simulink model "Link_A_org"  (Simulink 10.0)
settings: Solver=FixedStepAuto  StartTime=0  StopTime=15  FixedStep=1  RelTol=1e-3
StopFcn:
  | %set_param(gcb,'TAP_R_INI',[num2str(Tap_pu_R(end)), '  %Updated']);
libraries: simulink x9
(part 1 of 2)
settings Model: Creator=aw5670  LastModifiedBy=annonymous
settings DataIOCC: LimitDataPoints=on
settings OptimizationCC: BlockReduction=off  BooleanDataType=off
settings DebuggingCC: SaveWithParameterizedLinksMsg=none  SignalResolutionControl=TryResolveAllWithWarning
settings HardwareCC: TargetUnknown=on
settings GRTTargetCC: GeneratePreprocessorConditionals=Disable all  CombineOutputUpdateFcns=on  GRTInterface=off
settings ConfigComp: CovExternalEMLEnable=off  CovSFcnEnable=off

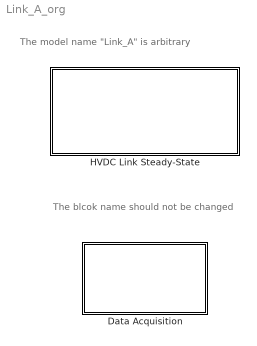
== system Link_A_org ==
  note: The blcok name should not be changed
  note: The model name "Link_A" is arbitrary
  Data Acquisition : Subsystem  mask{Ts=1}
      mask prompts: Ts "Sample time :"
      mask Display: disp('Open this block\nto visualize\nrecorded signals')
  HVDC Link Steady-State : Subsystem  mask(HVDC link steady-state model){NB_R=2, NOT_USED_3=, NOT_USED_4=, Pn_R=600, U1_R=[735, 0.0025, 0.01], U2_R=[200, 0.0025, 0.11], NOT_USED_0=DC current, NOT_USED_1=0, AMODE_ANGLE=5, LOCK_TAP_R=off, TCC_UDI0_MODE_R=off, ANGLE_R=[14.0, 17.0], Udi0_ref_R=280, TSTP_R=0.0125, TAP_R=[0.9375, 1.125], TAP_R_INI=0.9375  %Updated, Eac_R_INI=740.941  %Updated, NB_I=2, NOT_USED_5=, NOT_USED_6=, Pn_I=600, U1_I=[735, 0.0025, 0.01], U2_I=[200, 0.0025, 0.11], C_MODE_I=DC voltage, GAMMA_REF=22, VSCHED=500, GMODE_ANGLE=17, NOT_USED_2=0, LOCK_TAP_I=off, TCC_UDI0_MODE_I=off, ANGLE_I=[20.0, 23.0], Udi0_ref_I=280, TSTP_I=0.0125, TAP_I=[0.9125, 1.0875], TAP_I_INI=0.9875  %Updated, Eac_I_INI=759.4246  %Updated, RDC=12.0 + 2*0.3, RCOMP=0.3, MC_MODE=Power, SLACK_ST=Rectifier, SETVAL_MW=1000, SETVAL_kA=2, VCMODE=500*0.94, DELTI=0.2, Tap_pu_R=0.9375, Eac_R=740.8893, Udi0_R=290.4097, Tap_limited_R=0, alpha_R=16.1762, Idc_R=2, Vdc_R=524.6, Pdc_R=1049.2, Pac_R=1054.5333, Qac_R=479.4564, Tap_pu_I=0.975, Eac_I=758.8212, Udi0_I=285.9986, Tap_limited_I=0, alpha_I=144.587, gamma_I=22.8031, Vdc_I=499.4, Pdc_I=-998.8, Pac_I=-993.4667, Qac_I=562.6279, DC_iter=2, Ts=1}
      mask prompts: NB_R "Number of 6 pulse converter units in series"; NOT_USED_3 "AC bus name"; NOT_USED_4 "PQ load name"; Pn_R "Power (MVA)"; U1_R "Primary winding (AC side) parameters [V1 Ph-Ph(kVrms), R1(pu), L1(pu)]"; U2_R "Secondary winding (DC side) parameters [V2 Ph-Ph(kVrms), R2(pu), L2(pu)]"; NOT_USED_0 "Control mode"; NOT_USED_1 "not used"; AMODE_ANGLE "Minimum alpha (deg.)"; LOCK_TAP_R "Lock tap ratio"; TCC_UDI0_MODE_R "Udi0 control mode"; ANGLE_R "Angle range [min, max] (deg.)"; Udi0_ref_R "Udi0 reference (kV)"; TSTP_R "Tap step size (pu)"; TAP_R "Tap range [min, max] (pu)"; TAP_R_INI "Tap ratio (pu)"; Eac_R_INI "Primary AC voltage  (Ph-Ph(kVrms))"; NB_I "Number of 6 pulse converter units in series"; NOT_USED_5 "AC bus name"; NOT_USED_6 "PQ load name"; Pn_I "Power (MVA)"; U1_I "Primary winding (AC side) parameters [V1 Ph-Ph(kVrms), R1(pu), L1(pu)]"; U2_I "Secondary winding (DC side) parameters [V2 Ph-Ph(kVrms), R2(pu), L2(pu)]"; C_MODE_I "Control mode"; GAMMA_REF "Gamma reference (deg.)"; VSCHED "Voltage reference (kV)"; GMODE_ANGLE "Minimum gamma (deg.)"; NOT_USED_2 "Not used"; LOCK_TAP_I "Lock tap ratio"; TCC_UDI0_MODE_I "Udi0 control mode"; ANGLE_I "Angle range  [min, max] (deg.)"; Udi0_ref_I "Udi0 reference (kV)"; TSTP_I "Tap step size (pu)"; TAP_I "Tap range [min, max] (pu)"; TAP_I_INI "Tap ratio (pu)"; Eac_I_INI "Primary AC voltage  (Ph-Ph(kVrms))"; RDC "Total link resistance (ohm)"; RCOMP "Resistance between voltage measurement and converter (ohm)"; MC_MODE "Control mode"; SLACK_ST "Slack station"; SETVAL_MW "Power reference (MW)"; SETVAL_kA "Current reference (kA)"; VCMODE "Inverter DC voltage threshold in power control (kV)"; DELTI "Inverter current margin (kA)"; Tap_pu_R "Tap ratio (pu)"; Eac_R "Eac (kV)"; Udi0_R "Udi0 (kV)"; Tap_limited_R "Tap is limited"; alpha_R "Alpha (deg.)"; Idc_R "Idc (kA)"; Vdc_R "Vdc (kV)"; Pdc_R "Pdc (MW)"; Pac_R "Pac (MW)"; Qac_R "Qac (Mvar)"; Tap_pu_I "Tap ratio (pu)"; Eac_I "Eac (kV)"; Udi0_I "Udi0 (kV)"; Tap_limited_I "Tap is limited"; alpha_I "Alpha (deg.)"; gamma_I "Gamma (deg.)"; Vdc_I "Vdc (kV)"; Pdc_I "Pdc (MW)"; Pac_I "Pac (MW)"; Qac_I "Qac (Mvar)"; DC_iter "Iterations"; Ts "Sample time :"
      mask help: Implements a steady state model of a two terminal HVDC link for the DC load flow solution.
      mask init:
      | % History values 
      | Eac_R     = Eac_R_INI;
      | Eac_I     = Eac_I_INI;
      | TAPINI_R  = TAP_R_INI;
      | TAPINI_I  = TAP_I_INI;
      | 
      | % --- RECTIFIER ---
      | 
      | % Primary
      | V1_R = U1_R(1);
      | R1_R = U1_R(2);
      | L1_R = U1_R(3);
      | 
      | % Secondary
      | V2_R = U2_R(1);
      | R2_R = U2_R(2);
      | L2_R = U2_R(3);
      | 
      | % Nominal turn ratio (Usec/Uprim):
      | TR_R = V2_R/V1_R;
      | 
      | % Transformer reactance seen from secondary, per bridge [XC](ohm):
      | XC_R = (L1_R+L2_R)*V2_R^2/Pn_R;
      | 
      | % Transformer resistance seen from secondary, per bridge [RC](ohm):
      | RC_R = (R1_R+R2_R)* V2_R^2/Pn_R; 
      | 
      | % Tap Changer Control
      | ALFMIN_R=ANGLE_R(1);
      | ALFMAX_R=ANGLE_R(2);
      | 
      | TAPMN_R=TAP_R(1);
      | TAPMX_R=TAP_R(2);
      | 
      | % --- INVERTER ---
      | % Primary
      | V1_I = U1_I(1);
      | R1_I = U1_I(2);
      | L1_I = U1_I(3);
      | 
      | % Secondary
      | V2_I = U2_I(1);
      | R2_I = U2_I(2);
      | L2_I = U2_I(3);
      | 
      | % Nominal turn ratio (Usec/Uprim):
      | TR_I = V2_I/V1_I;
      | 
      | % Transformer reactance seen from secondary, per bridge [XC](ohm):
      | XC_I = (L1_I+L2_I)*V2_I^2/Pn_I;
      | 
      | % Transformer resistance seen from secondary, per bridge [RC](ohm):
      | RC_I = (R1_I+R2_I)* V2_I^2/Pn_I; 
      | 
      | % Pole Control
      | GC = C_MODE_I - 1;  % GC (0/1) is used in the model
      | 
      | % Tap Changer Control
      | GAMMIN_I=ANGLE_I(1);
      | GAMMAX_I=ANGLE_I(2);
      | 
      | TAPMN_I=TAP_I(1);
      | TAPMX_I=TAP_I(2);
      | 
      | DCVMIN_I   = VSCHED * (1 - TSTP_I);     %(kV)
      | DCVMAX_I   = VSCHED * (1 + TSTP_I);
      | 
      | %Udi0_min = (1-TSTP*0.75)* Udi0_ref;  % kV
      | %Udi0_max = (1+TSTP*0.75)* Udi0_ref;
      | 
      | % --- Master Control ---
      | MDC = MC_MODE - 1;     % MDC (0,1, or 2) used in the model 
      | 
      | if (MDC == 1)   
      |     SETVAL = SETVAL_MW;
      | elseif (MDC == 2)
      |     SETVAL = SETVAL_kA;
      | else
      |     SETVAL = 0;
      | end
      mask Help: web('HVDC_Link_SS_help.htm');
      mask TypeOptions NOT_USED_0: DC current
      mask Callback LOCK_TAP_R:
      | mode=get_param(gcb,'LOCK_TAP_R');
      | cb = get_param(gcb,'MaskEnables');
      | cb{11}='on'; cb{12}='on';
      | 
      | if strcmp(mode,'on')
      |  cb{11}='off';  % Udi0 control mode
      |  cb{12}='off';  % Angle range
      | end
      | 
      | set_param(gcb,'MaskEnables',cb);
      mask Callback TCC_UDI0_MODE_R:
      | mode=get_param(gcb,'TCC_UDI0_MODE_R');
      | cb = get_param(gcb,'MaskEnables');
      | cb{10}='on'; cb{12}='on'; cb{13}='off';
      | 
      | if strcmp(mode,'on')
      |  cb{12}='off';  % Angle range
      |  cb{10}='off';  % Lock the tap position
      |  cb{13}='on';  % Lock the tap position
      | end
      | 
      | set_param(gcb,'MaskEnables',cb);
      mask TypeOptions C_MODE_I: DC voltage | Gamma angle
      mask Callback C_MODE_I:
      | mode=get_param(gcb,'C_MODE_I');
      | cb = get_param(gcb,'MaskEnables');
      | cb{25}='on'; cb{26}='on'; cb{27}='on'; cb{31}='on';
      | 
      | if strcmp(mode,'Gamma angle')
      |  cb{26}='off';    % Voltage reference
      |  cb{27}='off';    % Minimum gamma
      |  cb{31}='off';    % Angle range (gamma_
      | else
      |  cb{25}='off';    % Gamma reference
      | end
      | 
      | set_param(gcb,'MaskEnables',cb);
      mask Callback LOCK_TAP_I:
      | mode=get_param(gcb,'LOCK_TAP_I');
      | cb = get_param(gcb,'MaskEnables');
      | cb{30}='on'; cb{31}='on';
      | 
      | if strcmp(mode,'on')
      |  cb{30}='off';  % Udi0 control mode
      |  cb{31}='off';  % Angle range
      | end
      | 
      | set_param(gcb,'MaskEnables',cb);
      mask Callback TCC_UDI0_MODE_I:
      | mode=get_param(gcb,'TCC_UDI0_MODE_I');
      | cb = get_param(gcb,'MaskEnables');
      | cb{29}='on'; cb{31}='on';  cb{32}='off';
      | 
      | if strcmp(mode,'on')
      |  cb{29}='off';  % Lock the tap position
      |  cb{31}='off';  % Angle range
      |  cb{32}='on';   % Udi0 reference
      | end
      | 
      | set_param(gcb,'MaskEnables',cb);
      mask TypeOptions MC_MODE: Blocked | Power | Current
      mask Callback MC_MODE:
      | mode=get_param(gcb,'MC_MODE');
      | cb = get_param(gcb,'MaskEnables');
      |  cb{40}='on'; cb{41}='on'; cb{42}='on'; cb{43}='on';
      | 
      | if strcmp(mode,'Current')
      |  cb{40}='off';     % Slack station
      |  cb{41}='off';     % Power reference
      |  cb{43}='off';     % Inverter DC ...
      | end
      | 
      | if strcmp(mode,'Power')
      |  cb{42}='off';     % Current reference
      | end
      | 
      | set_param(gcb,'MaskEnables',cb);
      | clear cb mode;
      mask TypeOptions SLACK_ST: Rectifier | Inverter
      mask DialogControl Update_tap_R Prompt: Update
      mask DialogControl Update_tap_R Callback:
      | set_param(gcb,'TAP_R_INI',[num2str(Tap_pu_R(end)), '  %Updated']);
      | 
      | % Reset output values
      | set_param(gcb,'Idc_R',[num2str(0)]);
      | set_param(gcb,'alpha_R',[num2str(0)]);
      | set_param(gcb,'Udi0_R',[num2str(0)]);
      | set_param(gcb,'Vdc_R',[num2str(0)]);
      | set_param(gcb,'Pac_R',[num2str(0)]);
      | set_param(gcb,'Qac_R',[num2str(0)]);
      | set_param(gcb,'Pdc_R',[num2str(0)]);
      mask DialogControl Update_tap_I Prompt: Update
      mask DialogControl Update_tap_I Callback:
      | set_param(gcb,'TAP_I_INI',[num2str(Tap_pu_I(end)), '  %Updated']);
      | 
      | % Reset output values
      | set_param(gcb,'gamma_I',[num2str(0)]);
      | set_param(gcb,'alpha_I',[num2str(0)]);
      | set_param(gcb,'Udi0_I',[num2str(0)]);
      | set_param(gcb,'Vdc_I',[num2str(0)]);
      | set_param(gcb,'Pdc_I',[num2str(0)]);
      | set_param(gcb,'Pac_I',[num2str(0)]);
      | set_param(gcb,'Qac_I',[num2str(0)]);
      mask DialogControl Container31 Prompt: Rectifier
      mask DialogControl Container33 Prompt: Inverter
      mask DialogControl Control4 Prompt: Compute and Update
      mask DialogControl Control4 Callback:
      | sim(gcs);
      | set_param(gcb,'DC_iter',[num2str(DC_iter(end))]);
      | % Rectifier
      | set_param(gcb,'Eac_R',[num2str(Eac_R(end))]);
      | set_param(gcb,'Tap_pu_R',[num2str(Tap_pu_R(end))]);
      | set_param(gcb,'Tap_limited_R',[num2str(Tap_limited_R(end))]);
      | set_param(gcb,'Idc_R',[num2str(Idc_R(end))]);
      | set_param(gcb,'alpha_R',[num2str(alpha_R(end))]);
      | set_param(gcb,'Udi0_R',[num2str(Udi0_R(end))]);
      | set_param(gcb,'Vdc_R',[num2str(Vdc_R(end))]);
      | set_param(gcb,'Pdc_R',[num2str(Pdc_R(end))]);
      | set_param(gcb,'Pac_R',[num2str(Pac_R(end))]);
      | set_param(gcb,'Qac_R',[num2str(Qac_R(end))]);
      | 
      | % Inverter
      | set_param(gcb,'Eac_I',[num2str(Eac_I(end))]);
      | set_param(gcb,'Tap_pu_I',[num2str(Tap_pu_I(end))]);
      | set_param(gcb,'Tap_limited_I',[num2str(Tap_limited_I(end))]);
      | set_param(gcb,'gamma_I',[num2str(gamma_I(end))]);
      | set_param(gcb,'alpha_I',[num2str(alpha_I(end))]);
      | set_param(gcb,'Udi0_I',[num2str(Udi0_I(end))]);
      | set_param(gcb,'Vdc_I',[num2str(Vdc_I(end))]);
      | set_param(gcb,'Pdc_I',[num2str(Pdc_I(end))]);
      | set_param(gcb,'Pac_I',[num2str(Pac_I(end))]);
      | set_param(gcb,'Qac_I',[num2str(Qac_I(end))]);
      mask Display: disp('Steady-state model\nof HVDC link\n\n(for DC load flow solution)')

== system Link_A_org/Data Acquisition ==
  note: Data acquisition
  Bus Selector : BusSelector  OutputSignals=Udi0
  Bus Selector1 : BusSelector  OutputSignals=Tap_pu,Tap_is_limited
  Bus Selector2 : BusSelector  OutputSignals=Tap_pu,Tap_is_limited
  Bus Selector3 : BusSelector  OutputSignals=alpha_deg,Qac,Pac,Eac
  Bus Selector4 : BusSelector  OutputSignals=Udi0,gamma_deg,Qac,Pac,Eac,alpha_deg
  Bus Selector6 : BusSelector  OutputSignals=Vdc_R,Vdc_I,Idc_R,Idc_I,Pdc_R,Pdc_I
  Bus Selector7 : BusSelector  OutputSignals=Io1,Io2
  DCLink : Scope  NumInputPorts=5
  INV : Scope  NumInputPorts=7
  Master : Scope  NumInputPorts=2
  REC : Scope  NumInputPorts=7
  Terminator : Terminator
  Terminator1 : Terminator
  wires:
  [m_TCC_R] -> Bus Selector2/1
  Bus Selector4/5 -> INV/7  "<Eac>"
  Bus Selector4/4 -> INV/6  "<Pac>"
  Bus Selector4/3 -> INV/5  "<Qac>"
  Bus Selector4/2 -> INV/4  "<gamma_deg>"
  Bus Selector4/1 -> INV/3  "<Udi0>"
  Bus Selector4/6 -> Terminator1/1  "<alpha_deg>"
  Bus Selector6/4 -> Terminator/1  "<Idc_I>"
  [m_dc_ntw] -> Bus Selector6/1
  [m_TCC_I] -> Bus Selector1/1
  [m_conv_I] -> Bus Selector4/1
  Bus Selector2/1 -> REC/1  "<Tap_pu>"
  Bus Selector6/1 -> DCLink/1  "<Vdc_R>"
  Bus Selector3/3 -> REC/6  "<Pac>"
  Bus Selector3/1 -> REC/4  "<alpha_deg>"
  Bus Selector3/2 -> REC/5  "<Qac>"
  [m_conv_R] -> Bus Selector3/1, Bus Selector/1
  Bus Selector/1 -> REC/3  "<Udi0>"
  [m_master] -> Bus Selector7/1
  Bus Selector7/1 -> Master/1  "<Io1>"
  Bus Selector7/2 -> Master/2  "<Io2>"
  Bus Selector2/2 -> REC/2  "<Tap_is_limited>"
  Bus Selector1/2 -> INV/2  "<Tap_is_limited>"
  Bus Selector6/2 -> DCLink/2  "<Vdc_I>"
  Bus Selector6/3 -> DCLink/3  "<Idc_R>"
  Bus Selector6/5 -> DCLink/4  "<Pdc_R>"
  Bus Selector6/6 -> DCLink/5  "<Pdc_I>"
  Bus Selector1/1 -> INV/1  "<Tap_pu>"
  Bus Selector3/4 -> REC/7  "<Eac>"

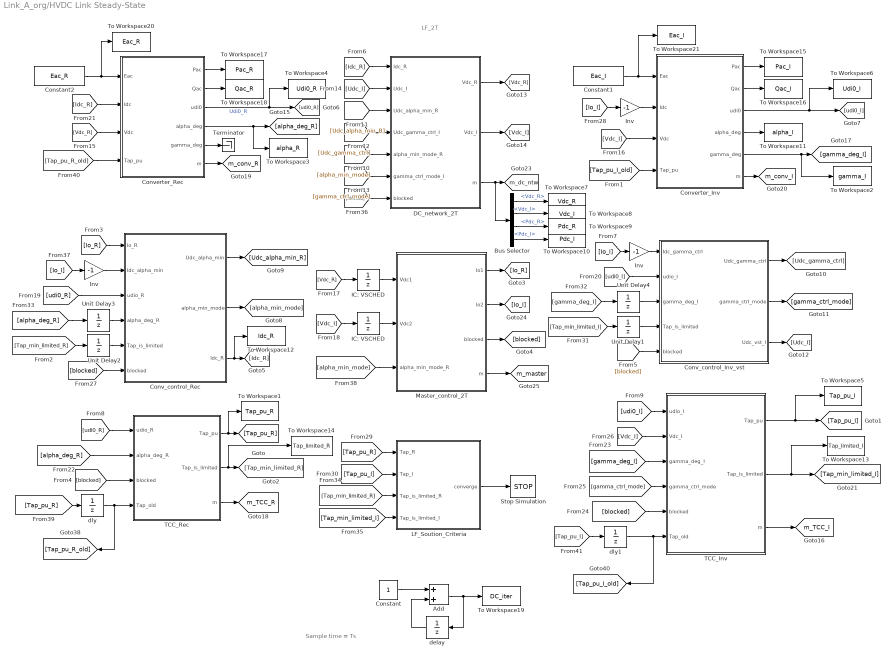
== system Link_A_org/HVDC Link Steady-State ==
  note: LF_2T
  note: Sample time = Ts
  " Inv " : Gain  Gain=-1
  Add : Sum
  Bus Selector : BusSelector  OutputSignals=Vdc_R,Vdc_I,Pdc_R,Pdc_I
  Constant : Constant
  Constant1 : Constant  Value=Eac_I
  Constant2 : Constant  Value=Eac_R
  Conv_control_Inv_vst : Subsystem  mask(Converter controls - voltage setting inverter){GC=GC, VSCHED=VSCHED, GMODE_ANGLE=GMODE_ANGLE, GAMMA_REF=GAMMA_REF, NB=NB_I, RC=RC_I, XC=XC_I}
      mask prompts: GC "Gamma control mode [GC] (1/0):"; VSCHED "Scheduled dc voltage [VSCHED] (kV):"; GMODE_ANGLE "Gamma minimum mode angle [GMODE_ANGLE] (deg):"; GAMMA_REF "Gamma reference angle [GAMMA_REF] (deg):"; NB "Number of 6 pulse bridges in series [NB]:"; RC "Resistance seen from secondary, per bridge [RC] (ohm):"; XC "Reactance seen from secondary, per bridge [XC] (ohm):"
  Conv_control_Rec : Subsystem  mask(Converter controls - Rectifier){AMODE_ANGLE=AMODE_ANGLE, NB=NB_R, RC=RC_R, XC=XC_R}
      mask prompts: AMODE_ANGLE "Alpha minimum mode angle   [AMODE_ANGLE] (deg):"; NB "Number of 6 pulse bridges in series [NB]:"; RC "Resistance seen from secondary, per bridge [RC] (ohm):"; XC "Reactance seen from secondary, per bridge [XC] (ohm):"
      settings: MinAlgLoopOccurrences=on
  Converter_Inv : Subsystem  mask(Converter unit data - Inverter){Pn=Pn_I, W1=[V1_I,  R1_I,  L1_I], W2=[V2_I, R2_I, L2_I], TR=V2_I/V1_I, RC=(R1_I+R2_I)* V2_I^2/Pn_I;, XC=(L1_I+L2_I)*V2_I^2/Pn_I;, NB=NB_I}
      mask prompts: Pn "One bridge, Transformer Nominal power [Pn(MVA)]:"; W1 "Primary winding (AC side) [V1 Ph-Ph(kVrms), R1(pu), L1(pu)]:"; W2 "Secondary winding (DC side) [V2 Ph-Ph(kVrms), R2 (pu), L2(pu)]:"; TR "Nominal turn ratio (Usec/Uprim) [TR] (pu):"; RC "Resistance seen from secondary, per bridge [RC] (ohm):"; XC "Reactance seen from secondary, per bridge [XC] (ohm):"; NB "Number of 6p bridges in series [NB]:"
  Converter_Rec : Subsystem  mask(Converter unit data - Rectifier){Pn=Pn_R, W1=[V1_R,  R1_R,  L1_R], W2=[V2_R,  R2_R,  L2_R], TR=V2_R/V1_R, RC=(R1_R+R2_R)* V2_R^2/Pn_R;, XC=(L1_R+L2_R)*V2_R^2/Pn_R;, NB=NB_R}
      mask prompts: Pn "One bridge, Transformer Nominal power [Pn(MVA)]:"; W1 "Primary winding (AC side) [V1 Ph-Ph(kVrms), R1(pu), L1(pu)]:"; W2 "Secondary winding (DC side) [V2 Ph-Ph(kVrms), R2 (pu), L2(pu)]:"; TR "Nominal turn ratio (Usec/Uprim) [TR] (pu):"; RC "Resistance seen from secondary, per bridge [RC] (ohm):"; XC "Reactance seen from secondary, per bridge [XC] (ohm):"; NB "Number of 6p bridges in series [NB]:"
  DC_network_2T : Subsystem  mask(DC network - 2 terminals){RDC=RDC, RCOMP=RCOMP}
      mask prompts: RDC "DC network resistance [RDC] (ohm):"; RCOMP "Compensating resistance for voltage control [RCOMP] (ohm):"
  IC: VSCHED : UnitDelay  InitialCondition=VSCHED  SampleTime=-1  HasFrameUpgradeWarning=on
  "IC: VSCHED " : UnitDelay  InitialCondition=VSCHED  SampleTime=-1  HasFrameUpgradeWarning=on
  "Inv " : Gain  Gain=-1
  "Inv  " : Gain  Gain=-1
  LF_Soution_Criteria : Subsystem
  Master_control_2T : Subsystem  mask(Master control for 3 terminals (RMCC)){MDC=MDC, SLACK_ST=SLACK_ST, SETVAL=SETVAL, VCMODE=VCMODE}
      mask prompts: MDC "Control mode [MDC] (0,1,2):"; SLACK_ST "Slack station [SLACK_ST] (1,2):"; SETVAL "Desired power or current [SETVAL] (MW or kA):"; VCMODE "Minimum DC voltage for power control [VCMODE] (kV):"
      mask help:
      | - The slack station (1, 2 or 3) will compensate for the DC network losses.
      | - Desired power or current: negative at inverter; positive at rectifier (sum shoud be zero).
  Stop Simulation : Stop
  TCC_Inv : Subsystem  mask(Tap Change Control (TCC) at the inverter){LOCK_TAP=LOCK_TAP_I, TCC_UDI0_MODE=TCC_UDI0_MODE_I, Udi0_ref=Udi0_ref_I, TAPINI=TAPINI_I, TAPMN=TAPMN_I, TAPMX=TAPMX_I, TSTP=TSTP_I, GAMMIN=GAMMIN_I, GAMMAX=GAMMAX_I, DCVMIN=DCVMIN_I, DCVMAX=DCVMAX_I}
      mask prompts: LOCK_TAP "Lock tap position at initial value [LOCK_TAP] (1/0):"; TCC_UDI0_MODE "TC in UDI0 control mode (around Udi0_ref) [TCC_UDI0_MODE] (1/0):"; Udi0_ref "Reference Udi0 voltage [Udi0_ref] (KV):"; TAPINI "Initial Tap ratio  [TAPINI] (pu):"; TAPMN "Minimum tap ratio [TAPMN] (pu):"; TAPMX "Maximum tap ratio [TAPMX] (pu):"; TSTP "Transformer tap-step [TSTP] (pu):"; GAMMIN "Minimum margin  (gamma) angle [GAMMIN] (deg):"; GAMMAX "Maximum margin  (gamma) angle [GAMMAX] (deg):"; DCVMIN "Minimum DC voltage [DCVMIN] (kV):"; DCVMAX "Maximum DC voltage [DCVMAX] (kV):"
      mask init:
      | Udi0_min = (1-TSTP*0.75)* Udi0_ref;  % kV
      | Udi0_max = (1+TSTP*0.75)* Udi0_ref;
      settings: AttributesFormatString=|
      | Udi0_min = (1-TSTP*0.75)* Udi0_ref
      | Udi0_max = (1+TSTP*0.75)* Udi0_ref
  TCC_Rec : Subsystem  mask(Tap Change Control (TCC) at the rectifier){LOCK_TAP=LOCK_TAP_R, TCC_UDI0_MODE=TCC_UDI0_MODE_R, Udi0_ref=Udi0_ref_R, TAPINI=TAPINI_R, TAPMN=TAPMN_R, TAPMX=TAPMX_R, TSTP=TSTP_R, ALFMIN=ALFMIN_R, ALFMAX=ALFMAX_R}
      mask prompts: LOCK_TAP "Lock tap position at initial value [LOCK_TAP] (1/0):"; TCC_UDI0_MODE "TC in UDI0 control mode (around Udi0_ref) [TCC_UDI0_MODE] (1/0):"; Udi0_ref "Reference Udi0 voltage [Udi0_ref] (KV):"; TAPINI "Initial Tap ratio  [TAPINI] (pu):"; TAPMN "Minimum tap ratio [TAPMN] (pu):"; TAPMX "Maximum tap ratio [TAPMX] (pu):"; TSTP "Transformer tap-step [TSTP] (pu):"; ALFMIN "Minimum firing (alpha) angle [ALFMIN] (deg):"; ALFMAX "Maximum firing (alpha) angle [ALFMAX] (deg):"
      mask init:
      | Udi0_min = (1-TSTP*0.75)* Udi0_ref;  % kV
      | Udi0_max = (1+TSTP*0.75)* Udi0_ref;
      settings: AttributesFormatString=|
      | Udi0_min = (1-TSTP*0.75)* Udi0_ref
      | Udi0_max = (1+TSTP*0.75)* Udi0_ref
  Terminator : Terminator
  To Workspace1 : ToWorkspace  VariableName=Tap_pu_R  SampleTime=-1
  To Workspace10 : ToWorkspace  VariableName=Pdc_I  SampleTime=-1
  To Workspace11 : ToWorkspace  VariableName=alpha_I  SampleTime=-1
  To Workspace12 : ToWorkspace  VariableName=Idc_R  SampleTime=-1
  To Workspace13 : ToWorkspace  VariableName=Tap_limited_I  SampleTime=-1
  To Workspace14 : ToWorkspace  VariableName=Tap_limited_R  SampleTime=-1
  To Workspace15 : ToWorkspace  VariableName=Pac_I  SampleTime=-1
  To Workspace16 : ToWorkspace  VariableName=Qac_I  SampleTime=-1
  To Workspace17 : ToWorkspace  VariableName=Pac_R  SampleTime=-1
  To Workspace18 : ToWorkspace  VariableName=Qac_R  SampleTime=-1
  To Workspace19 : ToWorkspace  VariableName=DC_iter  SampleTime=-1
  To Workspace2 : ToWorkspace  VariableName=gamma_I  SampleTime=-1
  To Workspace20 : ToWorkspace  VariableName=Eac_R  SampleTime=-1
  To Workspace21 : ToWorkspace  VariableName=Eac_I  SampleTime=-1
  To Workspace3 : ToWorkspace  VariableName=alpha_R  SampleTime=-1
  To Workspace4 : ToWorkspace  VariableName=Udi0_R  SampleTime=-1
  To Workspace5 : ToWorkspace  VariableName=Tap_pu_I  SampleTime=-1
  To Workspace6 : ToWorkspace  VariableName=Udi0_I  SampleTime=-1
  To Workspace7 : ToWorkspace  VariableName=Vdc_R  SampleTime=-1
  To Workspace8 : ToWorkspace  VariableName=Vdc_I  SampleTime=-1
  To Workspace9 : ToWorkspace  VariableName=Pdc_R  SampleTime=-1
  Unit Delay{1..4} (4 alike) : UnitDelay  SampleTime=-1  HasFrameUpgradeWarning=on
  delay : UnitDelay  SampleTime=Ts  HasFrameUpgradeWarning=on
      settings: AttributesFormatString=IC=%<InitialCondition>
  dly : UnitDelay  InitialCondition=TAPINI_R  SampleTime=-1  HasFrameUpgradeWarning=on
      settings: AttributesFormatString=IC=%<InitialCondition>
  dly1 : UnitDelay  InitialCondition=TAPINI_I  SampleTime=-1  HasFrameUpgradeWarning=on
      settings: AttributesFormatString=IC=%<InitialCondition>
  tag scope: m_TCC_I=global, m_TCC_R=global, m_conv_I=global, m_conv_R=global, m_dc_ntw=global, m_master=global
  wires:
  Constant1/1 -> Converter_Inv/1(Eac), To Workspace21/1
  Constant2/1 -> Converter_Rec/1(Eac), To Workspace20/1
  delay/1 -> Add/2
  Constant/1 -> Add/1
  Add/1 -> delay/1, To Workspace19/1
  [alpha_deg_R] -> TCC_Rec/2(alpha_deg_R)
  [Tap_pu_I] -> dly1/1
  dly1/1 -> TCC_Inv/6(Tap_old), [Tap_pu_I_old]
  [Tap_pu_R] -> dly/1
  dly/1 -> TCC_Rec/4(Tap_old), [Tap_pu_R_old]
  [gamma_deg_I] -> Unit Delay4/1
  Unit Delay4/1 -> Conv_control_Inv_vst/3(gamma_deg_I)
  Unit Delay3/1 -> Conv_control_Rec/4(alpha_deg_R)
  [alpha_deg_R] -> Unit Delay3/1
  Unit Delay2/1 -> Conv_control_Rec/5(Tap_is_limited)
  [Tap_min_limited_R] -> Unit Delay2/1
  Bus Selector/2 -> To Workspace8/1  "<Vdc_I>"
  Bus Selector/3 -> To Workspace9/1  "<Pdc_R>"
  Bus Selector/4 -> To Workspace10/1  "<Pdc_I>"
  Bus Selector/1 -> To Workspace7/1  "<Vdc_R>"
  [Tap_pu_I_old] -> Converter_Inv/4(Tap_pu)
  [Io_I] -> " Inv "/1
  [udi0_R] -> Conv_control_Rec/3(udio_R)
  [blocked] -> Conv_control_Rec/6(blocked)
  [blocked] -> DC_network_2T/7(blocked)
  [Tap_min_limited_I] -> LF_Soution_Criteria/4(Tap_is_limited_I)
  [Tap_min_limited_R] -> LF_Soution_Criteria/3(Tap_is_limited_R)
  [Tap_pu_I] -> LF_Soution_Criteria/2(Tap_I)
  TCC_Rec/3(m) -> [m_TCC_R]
  TCC_Rec/1(Tap_pu) -> [Tap_pu_R], To Workspace1/1
  TCC_Inv/3(m) -> [m_TCC_I]
  Unit Delay1/1 -> Conv_control_Inv_vst/4(Tap_is_limited)
  [blocked] -> Conv_control_Inv_vst/5(blocked)
  [Tap_min_limited_I] -> Unit Delay1/1
  Converter_Inv/2(Qac) -> To Workspace16/1
  Converter_Inv/1(Pac) -> To Workspace15/1
  Converter_Rec/2(Qac) -> To Workspace18/1
  Converter_Rec/1(Pac) -> To Workspace17/1
  [Tap_pu_R] -> LF_Soution_Criteria/1(Tap_R)
  Converter_Inv/6(m) -> [m_conv_I]
  Converter_Rec/6(m) -> [m_conv_R]
  [Vdc_I] -> Converter_Inv/3(Vdc)
  Converter_Rec/5(gamma_deg) -> Terminator/1
  [Vdc_I] -> TCC_Inv/2(Vdc_I)
  [gamma_ctrl_mode] -> TCC_Inv/4(gamma_ctrl_mode)
  [blocked] -> TCC_Inv/5(blocked)
  [gamma_deg_I] -> TCC_Inv/3(gamma_deg_I)
  Converter_Inv/5(gamma_deg) -> To Workspace2/1, [gamma_deg_I]
  Converter_Inv/4(alpha_deg) -> To Workspace11/1
  Converter_Rec/4(alpha_deg) -> [alpha_deg_R], To Workspace3/1
  [Idc_R] -> Converter_Rec/2(Idc)
  [udi0_I] -> Conv_control_Inv_vst/2(udio_I)
  [Vdc_I] -> "IC: VSCHED "/1
  [Vdc_R] -> IC: VSCHED/1
  [Vdc_R] -> Converter_Rec/3(Vdc)
  DC_network_2T/2(Vdc_I) -> [Vdc_I]
  DC_network_2T/1(Vdc_R) -> [Vdc_R]
  [Udc_I] -> DC_network_2T/2(Udc_I)
  Conv_control_Inv_vst/3(Udc_vst_I) -> [Udc_I]
  [gamma_ctrl_mode] -> DC_network_2T/6(gamma_ctrl_mode_I)
  Conv_control_Inv_vst/2(gamma_ctrl_mode) -> [gamma_ctrl_mode]
  [Udc_gamma_ctrl] -> DC_network_2T/4(Udc_gamma_ctrl_I)
  Conv_control_Inv_vst/1(Udc_gamma_ctrl) -> [Udc_gamma_ctrl]
  [Udc_alpha_min_R] -> DC_network_2T/3(Udc_alpha_min_R)
  Conv_control_Rec/1(Udc_alpha_min) -> [Udc_alpha_min_R]
  [alpha_min_mode] -> DC_network_2T/5(alpha_min_mode_R)
  Conv_control_Rec/2(alpha_min_mode) -> [alpha_min_mode]
  [Tap_pu_R_old] -> Converter_Rec/4(Tap_pu)
  [udi0_I] -> TCC_Inv/1(udio_I)
  [udi0_R] -> TCC_Rec/1(udio_R)
  Converter_Inv/3(udi0) -> [udi0_I], To Workspace6/1
  Converter_Rec/3(udi0) -> [udi0_R], To Workspace4/1  "Udi0_R"
  [Idc_R] -> DC_network_2T/1(Idc_R)
  [blocked] -> TCC_Rec/3(blocked)
  [Io_R] -> Conv_control_Rec/1(Io_R)
  TCC_Rec/2(Tap_is_limited) -> [Tap_min_limited_R], To Workspace14/1
  TCC_Inv/2(Tap_is_limited) -> [Tap_min_limited_I], To Workspace13/1
  TCC_Inv/1(Tap_pu) -> [Tap_pu_I], To Workspace5/1
  "IC: VSCHED "/1 -> Master_control_2T/2(Vdc2)
  IC: VSCHED/1 -> Master_control_2T/1(Vdc1)
  [alpha_min_mode] -> Master_control_2T/3(alpha_min_mode_R)
  Master_control_2T/1(Io1) -> [Io_R]
  Master_control_2T/2(Io2) -> [Io_I]
  Master_control_2T/3(blocked) -> [blocked]
  Master_control_2T/4(m) -> [m_master]
  "Inv "/1 -> Conv_control_Inv_vst/1(Idc_gamma_ctrl)
  [Io_I] -> "Inv "/1
  "Inv  "/1 -> Converter_Inv/2(Idc)
  [Io_I] -> "Inv  "/1
  DC_network_2T/3(m) -> [m_dc_ntw], Bus Selector/1
  " Inv "/1 -> Conv_control_Rec/2(Idc_alpha_min)
  Conv_control_Rec/3(Idc_R) -> [Idc_R], To Workspace12/1
  LF_Soution_Criteria/1(converge) -> Stop Simulation/1

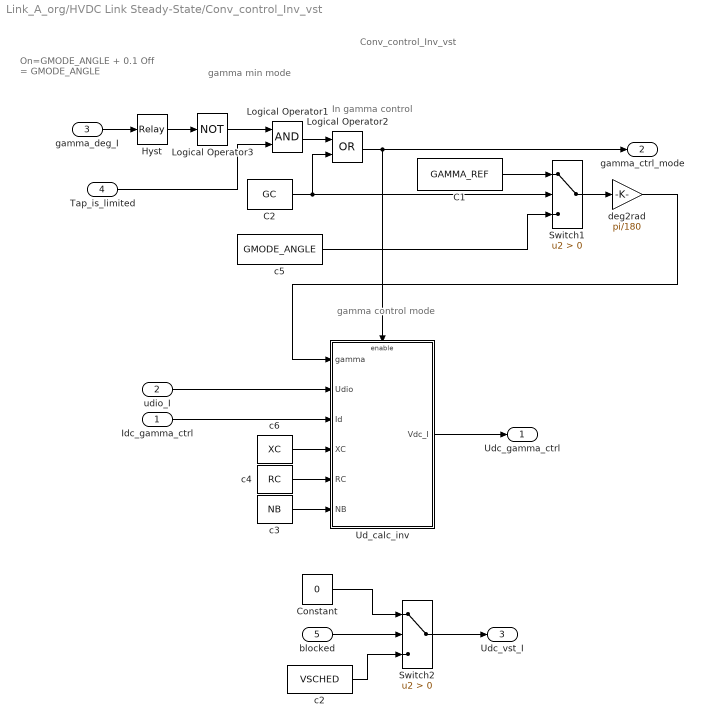
== system Link_A_org/HVDC Link Steady-State/Conv_control_Inv_vst ==
  note: gamma min mode
  note: On=GMODE_ANGLE + 0.1
      | Off = GMODE_ANGLE
  note: In gamma control
  note: gamma control mode
  note: Conv_control_Inv_vst
  Idc_gamma_ctrl : Inport
  udio_I : Inport  Port=2
  gamma_deg_I : Inport  Port=3
  Tap_is_limited : Inport  Port=4
  blocked : Inport  Port=5
  C1 : Constant  Value=GAMMA_REF
  C2 : Constant  Value=GC
  Constant : Constant  Value=0
  Hyst : Relay  OnSwitchValue=GMODE_ANGLE + 0.1  OffSwitchValue=GMODE_ANGLE
  Logical Operator1 : Logic  AllPortsSameDT=off  OutDataTypeStr=boolean
  Logical Operator2 : Logic  Operator=OR  AllPortsSameDT=off  OutDataTypeStr=boolean
  Logical Operator3 : Logic  Operator=NOT  AllPortsSameDT=off  OutDataTypeStr=boolean
  Switch1 : Switch  Criteria=u2 > Threshold
  Switch2 : Switch  Criteria=u2 > Threshold
  Ud_calc_inv : Subsystem
  c2 : Constant  Value=VSCHED
  c3 : Constant  Value=NB
  c4 : Constant  Value=RC
  c5 : Constant  Value=GMODE_ANGLE
  c6 : Constant  Value=XC
  deg2rad : Gain  Gain=pi/180
  Udc_gamma_ctrl : Outport
  gamma_ctrl_mode : Outport  Port=2
  Udc_vst_I : Outport  Port=3
  wires:
  Logical Operator3/1 -> Logical Operator1/1
  Hyst/1 -> Logical Operator3/1
  gamma_deg_I/1 -> Hyst/1
  Logical Operator2/1 -> gamma_ctrl_mode/1, Ud_calc_inv/Enable
  deg2rad/1 -> Ud_calc_inv/1(gamma)
  c5/1 -> Switch1/3
  C2/1 -> Logical Operator2/2, Switch1/2
  Logical Operator1/1 -> Logical Operator2/1
  c2/1 -> Switch2/3
  blocked/1 -> Switch2/2
  Constant/1 -> Switch2/1
  Switch2/1 -> Udc_vst_I/1
  Ud_calc_inv/1(Vdc_I) -> Udc_gamma_ctrl/1
  Idc_gamma_ctrl/1 -> Ud_calc_inv/3(Id)
  udio_I/1 -> Ud_calc_inv/2(Udio)
  c6/1 -> Ud_calc_inv/4(XC)
  c4/1 -> Ud_calc_inv/5(RC)
  c3/1 -> Ud_calc_inv/6(NB)
  C1/1 -> Switch1/1
  Switch1/1 -> deg2rad/1
  Tap_is_limited/1 -> Logical Operator1/2

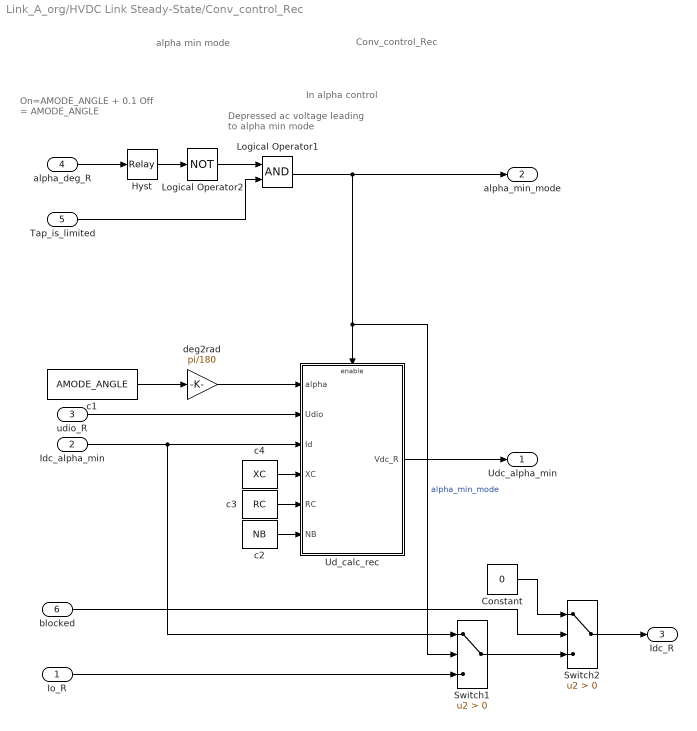
== system Link_A_org/HVDC Link Steady-State/Conv_control_Rec ==
  note: Depressed ac voltage
      |  leading to alpha min mode
  note: In alpha control
  note: Conv_control_Rec
  note: On=AMODE_ANGLE + 0.1
      | Off = AMODE_ANGLE
  note: alpha min mode
  Io_R : Inport
  Idc_alpha_min : Inport  Port=2
  udio_R : Inport  Port=3
  alpha_deg_R : Inport  Port=4
  Tap_is_limited : Inport  Port=5
  blocked : Inport  Port=6
  Constant : Constant  Value=0
  Hyst : Relay  OnSwitchValue=AMODE_ANGLE + 0.1  OffSwitchValue=AMODE_ANGLE
  Logical Operator1 : Logic  AllPortsSameDT=off  OutDataTypeStr=boolean
  Logical Operator2 : Logic  Operator=NOT  AllPortsSameDT=off  OutDataTypeStr=boolean
  Switch1 : Switch  Criteria=u2 > Threshold
  Switch2 : Switch  Criteria=u2 > Threshold
  Ud_calc_rec : Subsystem
  c1 : Constant  Value=AMODE_ANGLE
  c2 : Constant  Value=NB
  c3 : Constant  Value=RC
  c4 : Constant  Value=XC
  "deg2rad " : Gain  Gain=pi/180
  Udc_alpha_min : Outport
  alpha_min_mode : Outport  Port=2
  Idc_R : Outport  Port=3
  wires:
  Tap_is_limited/1 -> Logical Operator1/2
  Io_R/1 -> Switch1/3
  Logical Operator1/1 -> alpha_min_mode/1, Ud_calc_rec/Enable, Switch1/2  "alpha_min_mode"
  "deg2rad "/1 -> Ud_calc_rec/1(alpha)
  c1/1 -> "deg2rad "/1
  udio_R/1 -> Ud_calc_rec/2(Udio)
  c3/1 -> Ud_calc_rec/5(RC)
  c4/1 -> Ud_calc_rec/4(XC)
  alpha_deg_R/1 -> Hyst/1
  Ud_calc_rec/1(Vdc_R) -> Udc_alpha_min/1
  Idc_alpha_min/1 -> Ud_calc_rec/3(Id), Switch1/1
  Switch1/1 -> Switch2/3
  Switch2/1 -> Idc_R/1
  Constant/1 -> Switch2/1
  blocked/1 -> Switch2/2
  Hyst/1 -> Logical Operator2/1
  Logical Operator2/1 -> Logical Operator1/1
  c2/1 -> Ud_calc_rec/6(NB)

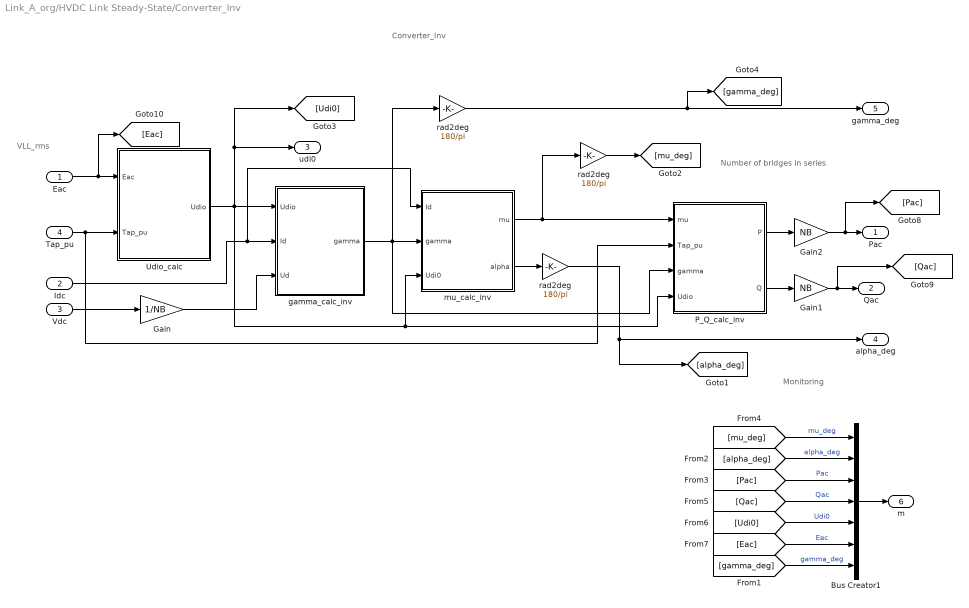
== system Link_A_org/HVDC Link Steady-State/Converter_Inv ==
  note: Monitoring
  note: Number of bridges in series
  note: VLL_rms
  note: Converter_Inv
  Eac : Inport
  Idc : Inport  Port=2
  Vdc : Inport  Port=3
  Tap_pu : Inport  Port=4
  Bus Creator1 : BusCreator  Inputs=7
  Gain : Gain  Gain=1/NB
  Gain1 : Gain  Gain=NB
  Gain2 : Gain  Gain=NB
  P_Q_calc_inv : Subsystem
  Udio_calc : Subsystem
  gamma_calc_inv : Subsystem
  mu_calc_inv : Subsystem
  "rad2deg " : Gain  Gain=180/pi
  "rad2deg  " : Gain  Gain=180/pi
  "rad2deg   " : Gain  Gain=180/pi
  Pac : Outport
  Qac : Outport  Port=2
  udi0 : Outport  Port=3
  alpha_deg : Outport  Port=4
  gamma_deg : Outport  Port=5
  m : Outport  Port=6
  wires:
  [Eac] -> Bus Creator1/6  "Eac"
  [gamma_deg] -> Bus Creator1/7  "gamma_deg"
  [Udi0] -> Bus Creator1/5  "Udi0"
  [Qac] -> Bus Creator1/4  "Qac"
  [Pac] -> Bus Creator1/3  "Pac"
  [alpha_deg] -> Bus Creator1/2  "alpha_deg"
  [mu_deg] -> Bus Creator1/1  "mu_deg"
  Bus Creator1/1 -> m/1
  "rad2deg   "/1 -> [alpha_deg], alpha_deg/1
  mu_calc_inv/2(alpha) -> "rad2deg   "/1
  mu_calc_inv/1(mu) -> "rad2deg  "/1, P_Q_calc_inv/1(mu)
  "rad2deg  "/1 -> [mu_deg]
  Gain1/1 -> [Qac], Qac/1
  Gain2/1 -> [Pac], Pac/1
  Gain/1 -> gamma_calc_inv/3(Ud)
  P_Q_calc_inv/1(P) -> Gain2/1
  P_Q_calc_inv/2(Q) -> Gain1/1
  "rad2deg "/1 -> [gamma_deg], gamma_deg/1
  gamma_calc_inv/1(gamma) -> P_Q_calc_inv/3(gamma), mu_calc_inv/2(gamma), "rad2deg "/1
  Vdc/1 -> Gain/1
  Idc/1 -> mu_calc_inv/1(Id), gamma_calc_inv/2(Id)
  Eac/1 -> [Eac], Udio_calc/1(Eac)
  Udio_calc/1(Udio) -> [Udi0], udi0/1, P_Q_calc_inv/4(Udio), mu_calc_inv/3(Udi0), gamma_calc_inv/1(Udio)
  Tap_pu/1 -> P_Q_calc_inv/2(Tap_pu), Udio_calc/2(Tap_pu)

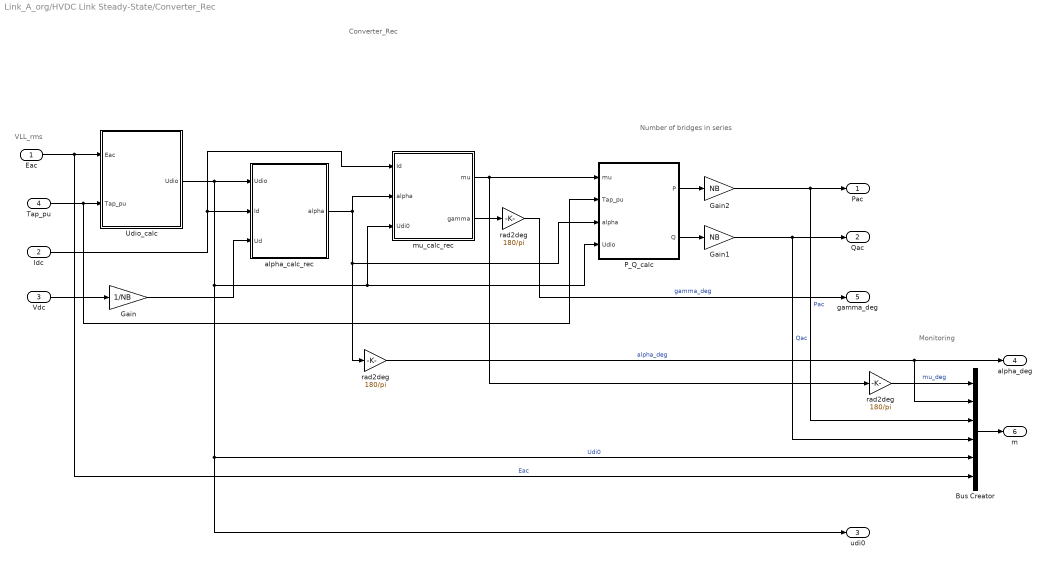
== system Link_A_org/HVDC Link Steady-State/Converter_Rec ==
  note: Converter_Rec
  note: VLL_rms
  note: Number of bridges in series
  note: Monitoring
  Eac : Inport
  Idc : Inport  Port=2
  Vdc : Inport  Port=3
  Tap_pu : Inport  Port=4
  Bus Creator : BusCreator  Inputs=6
  Gain : Gain  Gain=1/NB
  Gain1 : Gain  Gain=NB
  Gain2 : Gain  Gain=NB
  P_Q_calc : Subsystem
  Udio_calc : Subsystem
  alpha_calc_rec : Subsystem
  mu_calc_rec : Subsystem
  "rad2deg " : Gain  Gain=180/pi
  "rad2deg  " : Gain  Gain=180/pi
  "rad2deg   " : Gain  Gain=180/pi
  Pac : Outport
  Qac : Outport  Port=2
  udi0 : Outport  Port=3
  alpha_deg : Outport  Port=4
  gamma_deg : Outport  Port=5
  m : Outport  Port=6
  wires:
  Eac/1 -> Udio_calc/1(Eac), Bus Creator/6  "Eac"
  Udio_calc/1(Udio) -> udi0/1, Bus Creator/5, mu_calc_rec/3(Udi0), P_Q_calc/4(Udio), alpha_calc_rec/1(Udio)  "Udi0"
  Gain1/1 -> Bus Creator/4, Qac/1  "Qac"
  Gain2/1 -> Bus Creator/3, Pac/1  "Pac"
  "rad2deg "/1 -> Bus Creator/2, alpha_deg/1  "alpha_deg"
  "rad2deg  "/1 -> Bus Creator/1  "mu_deg"
  Tap_pu/1 -> P_Q_calc/2(Tap_pu), Udio_calc/2(Tap_pu)
  Idc/1 -> alpha_calc_rec/2(Id), mu_calc_rec/1(Id)
  Vdc/1 -> Gain/1
  alpha_calc_rec/1(alpha) -> "rad2deg "/1, P_Q_calc/3(alpha), mu_calc_rec/2(alpha)
  mu_calc_rec/1(mu) -> P_Q_calc/1(mu), "rad2deg  "/1
  mu_calc_rec/2(gamma) -> "rad2deg   "/1
  P_Q_calc/2(Q) -> Gain1/1
  P_Q_calc/1(P) -> Gain2/1
  Gain/1 -> alpha_calc_rec/3(Ud)
  Bus Creator/1 -> m/1
  "rad2deg   "/1 -> gamma_deg/1  "gamma_deg"

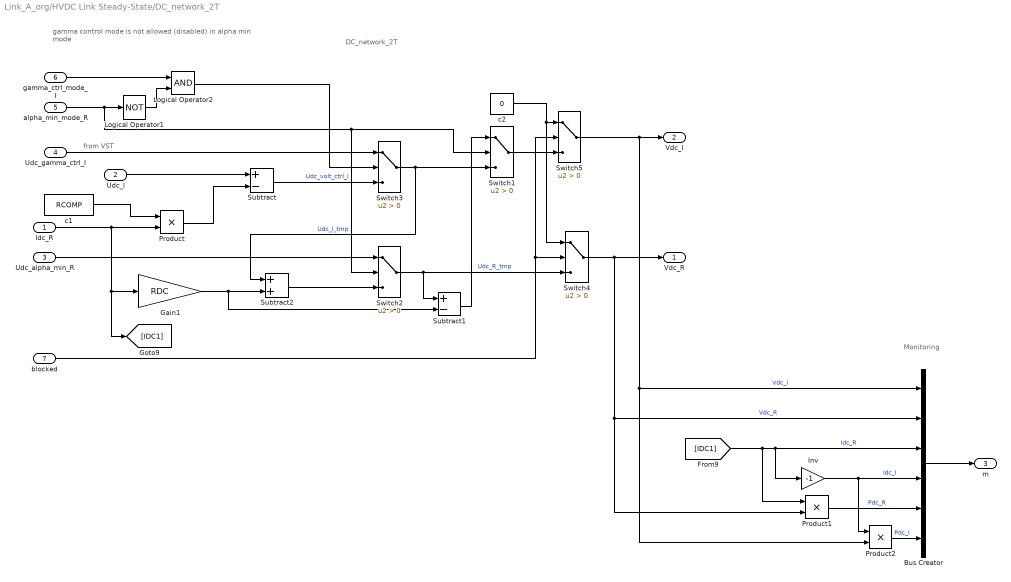
== system Link_A_org/HVDC Link Steady-State/DC_network_2T ==
  note: gamma control mode is not allowed (disabled)
      |  in alpha min mode
  note: DC_network_2T
  note: Monitoring
  note: from VST
  Idc_R : Inport
  Udc_I : Inport  Port=2
  Udc_alpha_min_R : Inport  Port=3
  Udc_gamma_ctrl_I : Inport  Port=4
  alpha_min_mode_R : Inport  Port=5
  gamma_ctrl_mode_I : Inport  Port=6
  blocked : Inport  Port=7
  Bus Creator : BusCreator  Inputs=6
  Gain1 : Gain  Gain=RDC
  Inv : Gain  Gain=-1
  Logical Operator1 : Logic  Operator=NOT  AllPortsSameDT=off  OutDataTypeStr=boolean
  Logical Operator2 : Logic  AllPortsSameDT=off  OutDataTypeStr=boolean
  Product : Product  RndMeth=Zero
  Product1 : Product  RndMeth=Zero
  Product2 : Product  RndMeth=Zero
  Subtract : Sum  Inputs=+-
  Subtract1 : Sum  Inputs=+-
  Subtract2 : Sum
  Switch{1..5} (5 alike) : Switch  Criteria=u2 > Threshold
  c1 : Constant  Value=RCOMP
  c2 : Constant  Value=0
  Vdc_R : Outport
  Vdc_I : Outport  Port=2
  m : Outport  Port=3
  wires:
  Product2/1 -> Bus Creator/6  "Pdc_I"
  [IDC1] -> Bus Creator/3, Inv/1, Product1/1  "Idc_R"
  Product1/1 -> Bus Creator/5  "Pdc_R"
  Inv/1 -> Product2/1, Bus Creator/4  "Idc_I"
  Logical Operator2/1 -> Switch3/2
  alpha_min_mode_R/1 -> Switch1/2, Switch2/2, Logical Operator1/1
  Logical Operator1/1 -> Logical Operator2/2
  gamma_ctrl_mode_I/1 -> Logical Operator2/1
  Udc_I/1 -> Subtract/1
  Idc_R/1 -> [IDC1], Gain1/1, Product/2
  Subtract/1 -> Switch3/3  "Udc_volt_ctrl_I"
  Udc_gamma_ctrl_I/1 -> Switch3/1
  Switch3/1 -> Switch1/3, Subtract2/1  "Udc_I_tmp"
  Gain1/1 -> Subtract2/2, Subtract1/2
  Subtract2/1 -> Switch2/3
  Udc_alpha_min_R/1 -> Switch2/1
  Switch2/1 -> Subtract1/1, Switch4/3  "Udc_R_tmp"
  Subtract1/1 -> Switch1/1
  Product/1 -> Subtract/2
  c1/1 -> Product/1
  Bus Creator/1 -> m/1
  Switch5/1 -> Bus Creator/1, Product2/2, Vdc_I/1  "Vdc_I"
  Switch4/1 -> Bus Creator/2, Product1/2, Vdc_R/1  "Vdc_R"
  Switch1/1 -> Switch5/3
  blocked/1 -> Switch4/2, Switch5/2
  c2/1 -> Switch5/1, Switch4/1

== system Link_A_org/HVDC Link Steady-State/LF_Soution_Criteria ==
  note: convergence criteria for DC LF solution
  Tap_R : Inport
  Tap_I : Inport  Port=2
  Tap_is_limited_R : Inport  Port=3
  Tap_is_limited_I : Inport  Port=4
  Abs : Abs
  Abs1 : Abs
  Compare To Constant : simulink/Logic and Bit Operations/Compare To Constant  relop=<=  const=1e-6  OutDataTypeStr=uint8
  Compare To Constant1 : simulink/Logic and Bit Operations/Compare To Constant  relop=<=  const=1e-6  OutDataTypeStr=uint8
  Difference : simulink/Discrete/Difference  ICPrevInput=0.0  InputProcessing=Inherited  OutMin=[]  OutMax=[]  OutDataType=fixdt(1, 16)  OutScaling=2^-10  DoSatur=off
  Difference1 : simulink/Discrete/Difference  ICPrevInput=0.0  InputProcessing=Inherited  OutMin=[]  OutMax=[]  OutDataType=fixdt(1, 16)  OutScaling=2^-10  DoSatur=off
  Logical Operator : Logic  AllPortsSameDT=off  OutDataTypeStr=boolean
  Logical Operator1 : Logic  AllPortsSameDT=off  OutDataTypeStr=boolean
  Logical Operator2 : Logic  Operator=NOT  AllPortsSameDT=off  OutDataTypeStr=boolean
  Logical Operator3 : Logic  Operator=OR  AllPortsSameDT=off  OutDataTypeStr=boolean
  Logical Operator4 : Logic  AllPortsSameDT=off  OutDataTypeStr=boolean
  Logical Operator5 : Logic  Operator=OR  AllPortsSameDT=off  OutDataTypeStr=boolean
  Logical Operator6 : Logic  Operator=NOT  AllPortsSameDT=off  OutDataTypeStr=boolean
  Unit Delay1 : UnitDelay  SampleTime=-1  HasFrameUpgradeWarning=on
  Unit Delay2 : UnitDelay  SampleTime=-1  HasFrameUpgradeWarning=on
  converge : Outport
  wires:
  Tap_I/1 -> Difference/1
  Tap_R/1 -> Difference1/1
  Difference1/1 -> Abs1/1
  Abs1/1 -> Compare To Constant1/1
  Abs/1 -> Compare To Constant/1
  Logical Operator/1 -> converge/1
  Difference/1 -> Abs/1
  Compare To Constant/1 -> Logical Operator1/1
  Tap_is_limited_I/1 -> Logical Operator2/1, Unit Delay2/1
  Logical Operator2/1 -> Logical Operator1/2
  Logical Operator1/1 -> Logical Operator3/1
  Logical Operator3/1 -> Logical Operator/2
  Unit Delay2/1 -> Logical Operator3/2
  Compare To Constant1/1 -> Logical Operator4/1
  Logical Operator4/1 -> Logical Operator5/1
  Tap_is_limited_R/1 -> Unit Delay1/1, Logical Operator6/1
  Logical Operator6/1 -> Logical Operator4/2
  Unit Delay1/1 -> Logical Operator5/2
  Logical Operator5/1 -> Logical Operator/1

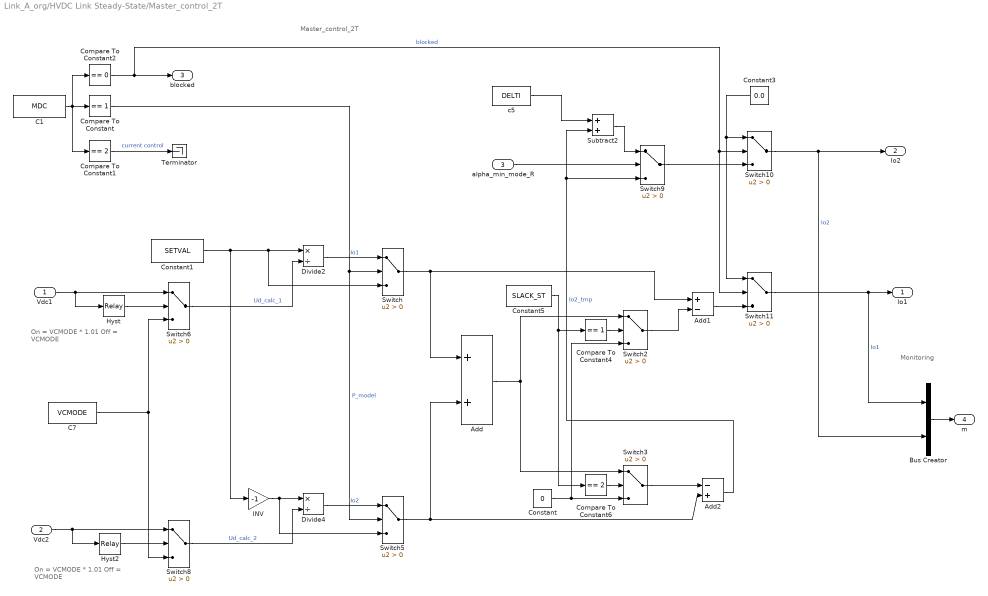
== system Link_A_org/HVDC Link Steady-State/Master_control_2T ==
  note: Master_control_2T
  note: On = VCMODE  * 1.01
      | Off = VCMODE
  note: On = VCMODE  * 1.01
      | Off = VCMODE
  note: Monitoring
  Vdc1 : Inport
  Vdc2 : Inport  Port=2
  alpha_min_mode_R : Inport  Port=3
  Add : Sum
  Add1 : Sum  Inputs=+-
  Add2 : Sum  Inputs=-+
  Bus Creator : BusCreator  Inputs=2
  C1 : Constant  Value=MDC
  C7 : Constant  Value=VCMODE
  Compare To Constant : simulink/Logic and Bit Operations/Compare To Constant  relop===  const=1  OutDataTypeStr=uint8  ZeroCross=off
  Compare To Constant1 : simulink/Logic and Bit Operations/Compare To Constant  relop===  const=2  OutDataTypeStr=uint8  ZeroCross=off
  Compare To Constant2 : simulink/Logic and Bit Operations/Compare To Constant  relop===  const=0  OutDataTypeStr=uint8  ZeroCross=off
  Compare To Constant4 : simulink/Logic and Bit Operations/Compare To Constant  relop===  const=1  OutDataTypeStr=uint8
  Compare To Constant6 : simulink/Logic and Bit Operations/Compare To Constant  relop===  const=2  OutDataTypeStr=uint8
  Constant : Constant  Value=0
  Constant1 : Constant  Value=SETVAL
  Constant3 : Constant  Value=0.0
  Constant5 : Constant  Value=SLACK_ST
  Divide2 : Product  Inputs=*/
  Divide4 : Product  Inputs=*/
  Hyst : Relay  OnSwitchValue=VCMODE*1.01  OffSwitchValue=VCMODE
  Hyst2 : Relay  OnSwitchValue=VCMODE*1.01  OffSwitchValue=VCMODE
  INV : Gain  Gain=-1
  Subtract2 : Sum
  Switch{,2..3,5..6,8..11} (9 alike) : Switch  Criteria=u2 > Threshold
  Terminator : Terminator
  c5 : Constant  Value=DELTI
  Io1 : Outport
  Io2 : Outport  Port=2
  blocked : Outport  Port=3
  m : Outport  Port=4
  wires:
  Switch10/1 -> Bus Creator/2, Io2/1  "Io2"
  Add1/1 -> Switch11/3
  Constant3/1 -> Switch11/1, Switch10/1
  Switch9/1 -> Switch10/3
  alpha_min_mode_R/1 -> Switch9/2
  Compare To Constant2/1 -> Switch11/2, Switch10/2, blocked/1  "blocked"
  C1/1 -> Compare To Constant1/1, Compare To Constant/1, Compare To Constant2/1
  Compare To Constant1/1 -> Terminator/1  "current control"
  Add/1 -> Switch2/1, Switch3/1
  Switch2/1 -> Add1/2
  INV/1 -> Divide4/1, Switch5/3
  Constant1/1 -> Divide2/1, Switch/3, INV/1
  Compare To Constant4/1 -> Switch2/2
  Compare To Constant6/1 -> Switch3/2
  Constant/1 -> Switch2/3, Switch3/3
  Constant5/1 -> Compare To Constant6/1, Compare To Constant4/1
  Divide2/1 -> Switch/1  "Io1"
  Divide4/1 -> Switch5/1  "Io2"
  Switch/1 -> Add/1, Add1/1
  Switch5/1 -> Add2/2, Add/2
  Compare To Constant/1 -> Switch/2, Switch5/2  "P_model"
  Switch3/1 -> Add2/1
  Hyst/1 -> Switch6/2
  C7/1 -> Switch6/3, Switch8/3
  Vdc1/1 -> Switch6/1, Hyst/1
  Hyst2/1 -> Switch8/2
  Vdc2/1 -> Switch8/1, Hyst2/1
  Switch6/1 -> Divide2/2  "Ud_calc_1"
  Switch8/1 -> Divide4/2  "Ud_calc_2"
  Bus Creator/1 -> m/1
  Add2/1 -> Subtract2/2, Switch9/3  "Io2_tmp"
  c5/1 -> Subtract2/1
  Subtract2/1 -> Switch9/1
  Switch11/1 -> Bus Creator/1, Io1/1  "Io1"

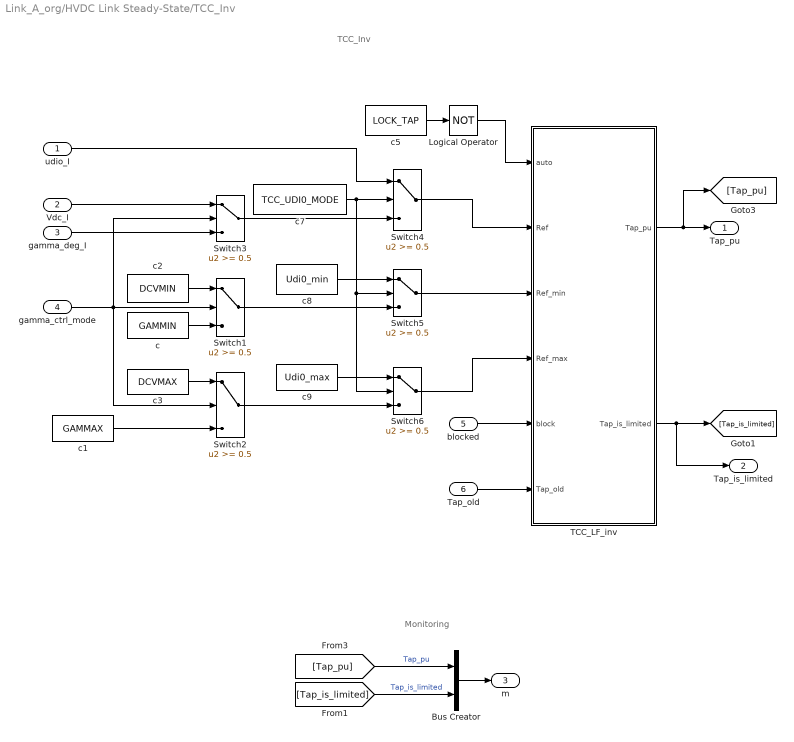
== system Link_A_org/HVDC Link Steady-State/TCC_Inv ==
  note: Monitoring
  note: TCC_Inv
  udio_I : Inport
  Vdc_I : Inport  Port=2
  gamma_deg_I : Inport  Port=3
  gamma_ctrl_mode : Inport  Port=4
  blocked : Inport  Port=5
  Tap_old : Inport  Port=6
  Bus Creator : BusCreator  Inputs=2
  Logical Operator : Logic  Operator=NOT  AllPortsSameDT=off  OutDataTypeStr=boolean
  Switch{1..6} (6 alike) : Switch  Threshold=0.5
  TCC_LF_inv : Subsystem
  c : Constant  Value=GAMMIN
  c1 : Constant  Value=GAMMAX
  c2 : Constant  Value=DCVMIN
  c3 : Constant  Value=DCVMAX
  c5 : Constant  Value=LOCK_TAP
  c7 : Constant  Value=TCC_UDI0_MODE
  c8 : Constant  Value=Udi0_min
  c9 : Constant  Value=Udi0_max
  Tap_pu : Outport
  Tap_is_limited : Outport  Port=2
  m : Outport  Port=3
  wires:
  [Tap_is_limited] -> Bus Creator/2  "Tap_is_limited"
  [Tap_pu] -> Bus Creator/1  "Tap_pu"
  Bus Creator/1 -> m/1
  Vdc_I/1 -> Switch3/1
  c2/1 -> Switch1/1
  c3/1 -> Switch2/1
  gamma_deg_I/1 -> Switch3/3
  c1/1 -> Switch2/3
  c/1 -> Switch1/3
  gamma_ctrl_mode/1 -> Switch3/2, Switch2/2, Switch1/2
  blocked/1 -> TCC_LF_inv/5(block)
  c5/1 -> Logical Operator/1
  Logical Operator/1 -> TCC_LF_inv/1(auto)
  udio_I/1 -> Switch4/1
  c7/1 -> Switch4/2, Switch5/2, Switch6/2
  c8/1 -> Switch5/1
  c9/1 -> Switch6/1
  Switch3/1 -> Switch4/3
  Switch1/1 -> Switch5/3
  Switch2/1 -> Switch6/3
  Switch4/1 -> TCC_LF_inv/2(Ref)
  Switch5/1 -> TCC_LF_inv/3(Ref_min)
  Switch6/1 -> TCC_LF_inv/4(Ref_max)
  Tap_old/1 -> TCC_LF_inv/6(Tap_old)
  TCC_LF_inv/2(Tap_is_limited) -> [Tap_is_limited], Tap_is_limited/1
  TCC_LF_inv/1(Tap_pu) -> [Tap_pu], Tap_pu/1

== system Link_A_org/HVDC Link Steady-State/TCC_Rec ==
  note: TCC_Rec
  note: Monitoring
  udio_R : Inport
  alpha_deg_R : Inport  Port=2
  blocked : Inport  Port=3
  Tap_old : Inport  Port=4
  Bus Creator : BusCreator  Inputs=2
  Logical Operator : Logic  Operator=NOT  AllPortsSameDT=off  OutDataTypeStr=boolean
  Switch4 : Switch  Threshold=0.5
  Switch5 : Switch  Threshold=0.5
  Switch6 : Switch  Threshold=0.5
  TCC_LF : Subsystem
  c1 : Constant  Value=ALFMAX
  c2 : Constant  Value=ALFMIN
  c5 : Constant  Value=LOCK_TAP
  c7 : Constant  Value=TCC_UDI0_MODE
  c8 : Constant  Value=Udi0_min
  c9 : Constant  Value=Udi0_max
  Tap_pu : Outport
  Tap_is_limited : Outport  Port=2
  m : Outport  Port=3
  wires:
  Tap_old/1 -> TCC_LF/6(Tap_old)
  blocked/1 -> TCC_LF/5(block)
  c5/1 -> Logical Operator/1
  Logical Operator/1 -> TCC_LF/1(auto)
  udio_R/1 -> Switch4/1
  c7/1 -> Switch6/2, Switch5/2, Switch4/2
  c8/1 -> Switch5/1
  c9/1 -> Switch6/1
  alpha_deg_R/1 -> Switch4/3
  c1/1 -> Switch6/3
  Switch4/1 -> TCC_LF/2(Ref)
  Switch5/1 -> TCC_LF/3(Ref_min)
  Switch6/1 -> TCC_LF/4(Ref_max)
  c2/1 -> Switch5/3
  Bus Creator/1 -> m/1
  TCC_LF/1(Tap_pu) -> Bus Creator/1, Tap_pu/1  "Tap_pu"
  TCC_LF/2(Tap_is_limited) -> Bus Creator/2, Tap_is_limited/1  "Tap_is_limited"

== system Link_A_org/HVDC Link Steady-State/Conv_control_Inv_vst/Ud_calc_inv ==
  note: Equivalent commtating resistance
  note: 3/pi
  note: Udio * cos(gamma)
  note: Ud_calc_inv
  note: Transformer windings & Thyristor
      |  resistance drop
  gamma : Inport
  Udio : Inport  Port=2
  Id : Inport  Port=3
  XC : Inport  Port=4
  RC : Inport  Port=5
  NB : Inport  Port=6
  Enable (held) : EnablePort  PropagateVarSize=During execution
  Gain1 : Gain  Gain=2
  Gain2 : Gain  Gain=3/pi
  Product{1..4} (4 alike) : Product  RndMeth=Zero
  Subtract : Sum  Inputs=+-+
  Trigonometric Function : Trigonometry  Operator=cos
  Vdc_I : Outport
  wires:
  gamma/1 -> Trigonometric Function/1
  Trigonometric Function/1 -> Product1/2
  Udio/1 -> Product1/1
  Product1/1 -> Subtract/1  "udio_cos_gamma"
  Id/1 -> Product2/1, Product4/1
  Product2/1 -> Subtract/2  "RcId"
  Gain2/1 -> Product2/2
  RC/1 -> Gain1/1
  Gain1/1 -> Product4/2
  Product4/1 -> Subtract/3
  XC/1 -> Gain2/1
  Subtract/1 -> Product3/1
  Product3/1 -> Vdc_I/1
  NB/1 -> Product3/2

== system Link_A_org/HVDC Link Steady-State/Conv_control_Rec/Ud_calc_rec ==
  note: Equivalent commtating resistance
  note: 3/pi
  note: Udio * cos(alpha)
  note: Ud_calc_rec
  note: Transformer windings & Thyristor
      |  resistance drop
  alpha : Inport
  Udio : Inport  Port=2
  Id : Inport  Port=3
  XC : Inport  Port=4
  RC : Inport  Port=5
  NB : Inport  Port=6
  Enable (held) : EnablePort  PropagateVarSize=During execution
  Gain1 : Gain  Gain=2
  Gain2 : Gain  Gain=3/pi
  Product{1..4} (4 alike) : Product  RndMeth=Zero
  Subtract : Sum  Inputs=+--
  Trigonometric Function : Trigonometry  Operator=cos
  Vdc_R : Outport
  wires:
  alpha/1 -> Trigonometric Function/1
  Trigonometric Function/1 -> Product1/2
  Udio/1 -> Product1/1
  Product1/1 -> Subtract/1  "udio_cos_alpha"
  Id/1 -> Product2/1, Product4/1
  Product2/1 -> Subtract/2  "RcId"
  Gain2/1 -> Product2/2
  RC/1 -> Gain1/1
  Gain1/1 -> Product4/2
  Product4/1 -> Subtract/3
  XC/1 -> Gain2/1
  Subtract/1 -> Product3/1
  Product3/1 -> Vdc_R/1
  NB/1 -> Product3/2

== system Link_A_org/HVDC Link Steady-State/Converter_Inv/P_Q_calc_inv ==
  note: Negative in inverter
      |  (gamma)
  mu : Inport
  Tap_pu : Inport  Port=2
  gamma : Inport  Port=3
  Udio : Inport  Port=4
  "Avoid zero " : Saturate  UpperLimit=inf  LowerLimit=eps
  Gain1 : Gain  Gain=NB
  Gain2 : Gain  Gain=NB
  Gain3 : Gain  Gain=-1
  Id_Iq_Pq_calc : Subsystem
  Terminator : Terminator
  Terminator1 : Terminator
  P : Outport
  Q : Outport  Port=2
  wires:
  Gain1/1 -> Terminator1/1
  Gain2/1 -> Terminator/1
  Id_Iq_Pq_calc/4(P_q) -> Q/1
  Id_Iq_Pq_calc/3(P_d) -> Gain3/1
  Udio/1 -> Id_Iq_Pq_calc/1(Udio)
  "Avoid zero "/1 -> Id_Iq_Pq_calc/2(Tap_pu)
  Tap_pu/1 -> "Avoid zero "/1
  mu/1 -> Id_Iq_Pq_calc/3(mu)
  gamma/1 -> Id_Iq_Pq_calc/4(angle)
  Id_Iq_Pq_calc/1(I_d) -> Gain2/1
  Id_Iq_Pq_calc/2(I_q) -> Gain1/1
  Gain3/1 -> P/1

== system Link_A_org/HVDC Link Steady-State/Converter_Inv/Udio_calc ==
  note: Udio_calc
  note: 3*sqrt(2)/pi * Usec_nom/Uprim_nom
  note: VLL_rms
  Eac : Inport
  Tap_pu : Inport  Port=2
  "Avoid zero " : Saturate  UpperLimit=inf  LowerLimit=eps
  Divide3 : Product  Inputs=*/
  k : Gain  Gain=(3*sqrt(2)/pi) * TR
  Udio : Outport
  wires:
  Divide3/1 -> Udio/1
  Tap_pu/1 -> "Avoid zero "/1
  "Avoid zero "/1 -> Divide3/2
  Eac/1 -> k/1
  k/1 -> Divide3/1

== system Link_A_org/HVDC Link Steady-State/Converter_Inv/gamma_calc_inv ==
  note: Equivalent commtating resistance (Rc)
  note: 3/pi
  note: gamma_calc_inv
  note: Transformer windings resistance drop
  Udio : Inport
  Id : Inport  Port=2
  Ud : Inport  Port=3
  Avoid zero : Saturate  UpperLimit=inf  LowerLimit=eps
  Divide : Product  Inputs=*/
  Gain1 : Gain  Gain=2
  Gain2 : Gain  Gain=3/pi
  Min:-1 Max:1 : Saturate  UpperLimit=1.0  LowerLimit=-1.0
  Product2 : Product  RndMeth=Zero
  Product4 : Product  RndMeth=Zero
  Subtract : Sum  Inputs=++-
  Trigonometric Function1 : Trigonometry  Operator=acos
  c : Constant  Value=XC
  c3 : Constant  Value=RC
  gamma : Outport
  wires:
  Id/1 -> Product2/1, Product4/1
  Product2/1 -> Subtract/2  "RcId"
  Gain2/1 -> Product2/2  "Rc"
  Product4/1 -> Subtract/3
  Ud/1 -> Subtract/1
  Subtract/1 -> Divide/1
  Udio/1 -> Avoid zero/1
  Avoid zero/1 -> Divide/2
  Divide/1 -> Min:-1 Max:1/1
  c3/1 -> Gain1/1
  Gain1/1 -> Product4/2
  Trigonometric Function1/1 -> gamma/1
  c/1 -> Gain2/1
  Min:-1 Max:1/1 -> Trigonometric Function1/1

== system Link_A_org/HVDC Link Steady-State/Converter_Inv/mu_calc_inv ==
  note: Uac_sec_LL_rms / sqrt(2)
  note: pi/6
  note: mu_calc_inv
  note: mu = arcos( cos (gamma - 2 (Xc*3/pi*Id/ Udio)) - gamma
  note: alpha = pi - gamma - mu
  Id : Inport
  gamma : Inport  Port=2
  Udi0 : Inport  Port=3
  Avoid zero : Saturate  UpperLimit=inf  LowerLimit=eps
  Constant : Constant  Value=pi
  Divide1 : Product  Inputs=*/
  Divide2 : Product  Inputs=*/
  Gain2 : Gain  Gain=pi/6
  Min=-1 Max=1 : Saturate  UpperLimit=1  LowerLimit=-1
  Subtract1 : Sum  Inputs=+-
  Subtract2 : Sum  Inputs=+-
  Subtract3 : Sum  Inputs=--+
  Trigonometric Function : Trigonometry  Operator=acos
  Trigonometric Function1 : Trigonometry  Operator=cos
  c : Constant  Value=XC
  mu : Outport
  alpha : Outport  Port=2
  wires:
  Trigonometric Function1/1 -> Subtract1/1
  Subtract3/1 -> alpha/1
  Divide2/1 -> Avoid zero/1  "Is2"
  Gain2/1 -> Divide2/1
  Udi0/1 -> Gain2/1
  Subtract2/1 -> mu/1, Subtract3/1
  gamma/1 -> Trigonometric Function1/1, Subtract3/2, Subtract2/2
  Trigonometric Function/1 -> Subtract2/1
  Subtract1/1 -> Min=-1 Max=1/1
  Divide1/1 -> Subtract1/2
  Avoid zero/1 -> Divide1/2
  Id/1 -> Divide1/1
  c/1 -> Divide2/2
  Min=-1 Max=1/1 -> Trigonometric Function/1
  Constant/1 -> Subtract3/3

== system Link_A_org/HVDC Link Steady-State/Converter_Rec/P_Q_calc ==
  note: P_Q_calc
  mu : Inport
  Tap_pu : Inport  Port=2
  alpha : Inport  Port=3
  Udio : Inport  Port=4
  "Avoid zero " : Saturate  UpperLimit=inf  LowerLimit=eps
  Gain1 : Gain  Gain=NB
  Gain2 : Gain  Gain=NB
  Id_Iq_Pq_calc : Subsystem
  Terminator : Terminator
  Terminator1 : Terminator
  P : Outport
  Q : Outport  Port=2
  wires:
  Id_Iq_Pq_calc/2(I_q) -> Gain1/1
  Id_Iq_Pq_calc/1(I_d) -> Gain2/1
  alpha/1 -> Id_Iq_Pq_calc/4(angle)
  mu/1 -> Id_Iq_Pq_calc/3(mu)
  Tap_pu/1 -> "Avoid zero "/1
  "Avoid zero "/1 -> Id_Iq_Pq_calc/2(Tap_pu)
  Udio/1 -> Id_Iq_Pq_calc/1(Udio)
  Id_Iq_Pq_calc/3(P_d) -> P/1
  Id_Iq_Pq_calc/4(P_q) -> Q/1
  Gain2/1 -> Terminator/1
  Gain1/1 -> Terminator1/1

== system Link_A_org/HVDC Link Steady-State/Converter_Rec/Udio_calc ==
  note: VLL_rms
  note: 3*sqrt(2)/pi * Usec_nom/Uprim_nom
  note: Udio_calc
  Eac : Inport
  Tap_pu : Inport  Port=2
  "Avoid zero " : Saturate  UpperLimit=inf  LowerLimit=eps
  Divide3 : Product  Inputs=*/
  k : Gain  Gain=(3*sqrt(2)/pi) * TR
  Udio : Outport
  wires:
  k/1 -> Divide3/1
  Eac/1 -> k/1
  "Avoid zero "/1 -> Divide3/2
  Tap_pu/1 -> "Avoid zero "/1
  Divide3/1 -> Udio/1
